simulink library "threeTethers_cl"  (R2018b)
settings: Solver=VariableStepAuto  StartTime=0.0  StopTime=10.0  RelTol=1e-3
undefined symbols (not defined in the file): gnd_station, ini_euler_ang, ini_Rcm_o, R11_g, R1n_cm, R21_g, R2n_cm, R31_g, R3n_cm, rotation_sequence, sim_param
libraries: singleTether_cl x3
settings Model: Creator=mcobb  LastModifiedBy=mcobb

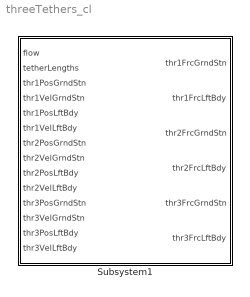
== system threeTethers_cl ==
  Subsystem1 : Subsystem

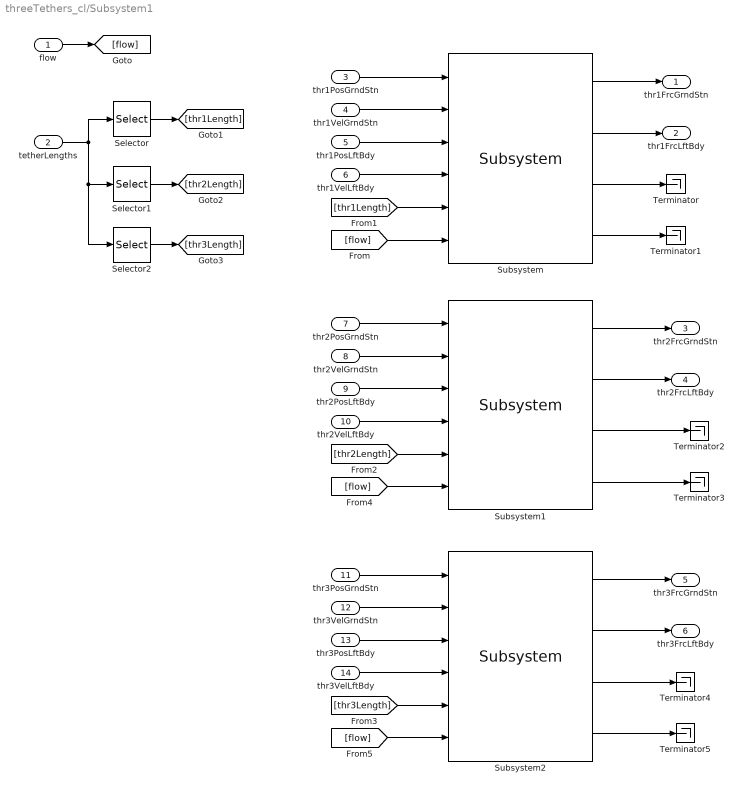
== system threeTethers_cl/Subsystem1 ==
  flow : Inport
  tetherLengths : Inport  Port=2
  thr1PosGrndStn : Inport  Port=3
  thr1VelGrndStn : Inport  Port=4
  thr1PosLftBdy : Inport  Port=5
  thr1VelLftBdy : Inport  Port=6
  thr2PosGrndStn : Inport  Port=7
  thr2VelGrndStn : Inport  Port=8
  thr2PosLftBdy : Inport  Port=9
  thr2VelLftBdy : Inport  Port=10
  thr3PosGrndStn : Inport  Port=11
  thr3VelGrndStn : Inport  Port=12
  thr3PosLftBdy : Inport  Port=13
  thr3VelLftBdy : Inport  Port=14
  Selector : Selector  InputPortWidth=3  IndexOptions=Index vector (dialog)  Indices=1  OutputSizes=1
  Selector1 : Selector  InputPortWidth=3  IndexOptions=Index vector (dialog)  Indices=1  OutputSizes=1
  Selector2 : Selector  InputPortWidth=3  IndexOptions=Index vector (dialog)  Indices=1  OutputSizes=1
  Subsystem : singleTether_cl/Subsystem  N=sim_param.N  dia_t=sim_param.tether_param.tether_diameter(1)  E=sim_param.tether_param.tether_youngs  rho_tether=sim_param.tether_param.tether_density+ sim_param.env_param.density  Cd=sim_param.tether_param.CD_cylinder  zeta=sim_param.tether_param.damping_ratio  rho=sim_param.env_param.density  mass=sim_param.geom_param.mass  ini_Rn_o=ini_Rcm_o + rotation_sequence(ini_euler_ang)*R1n_cm  ini_R1_o=gnd_station + R11_g
  Subsystem1 : singleTether_cl/Subsystem  N=sim_param.N  dia_t=sim_param.tether_param.tether_diameter(2)  E=sim_param.tether_param.tether_youngs  rho_tether=sim_param.tether_param.tether_density+ sim_param.env_param.density  Cd=sim_param.tether_param.CD_cylinder  zeta=sim_param.tether_param.damping_ratio  rho=sim_param.env_param.density  mass=sim_param.geom_param.mass  ini_Rn_o=ini_Rcm_o + rotation_sequence(ini_euler_ang)*R2n_cm  ini_R1_o=gnd_station + R21_g
  Subsystem2 : singleTether_cl/Subsystem  N=sim_param.N  dia_t=sim_param.tether_param.tether_diameter(3)  E=sim_param.tether_param.tether_youngs  rho_tether=sim_param.tether_param.tether_density+ sim_param.env_param.density  Cd=sim_param.tether_param.CD_cylinder  zeta=sim_param.tether_param.damping_ratio  rho=sim_param.env_param.density  mass=sim_param.geom_param.mass  ini_Rn_o=ini_Rcm_o + rotation_sequence(ini_euler_ang)*R3n_cm  ini_R1_o=gnd_station + R31_g
  Terminator{,1..5} (6 alike) : Terminator
  thr1FrcGrndStn : Outport
  thr1FrcLftBdy : Outport  Port=2
  thr2FrcGrndStn : Outport  Port=3
  thr2FrcLftBdy : Outport  Port=4
  thr3FrcGrndStn : Outport  Port=5
  thr3FrcLftBdy : Outport  Port=6
  wires:
  thr1PosGrndStn/1 -> Subsystem/1
  thr1VelGrndStn/1 -> Subsystem/2
  thr1VelLftBdy/1 -> Subsystem/4
  thr1PosLftBdy/1 -> Subsystem/3
  flow/1 -> [flow]
  [flow] -> Subsystem/6
  Selector/1 -> [thr1Length]
  tetherLengths/1 -> Selector/1, Selector1/1, Selector2/1
  Selector1/1 -> [thr2Length]
  Selector2/1 -> [thr3Length]
  [thr1Length] -> Subsystem/5
  [thr2Length] -> Subsystem1/5
  [thr3Length] -> Subsystem2/5
  [flow] -> Subsystem1/6
  [flow] -> Subsystem2/6
  thr2PosGrndStn/1 -> Subsystem1/1
  thr2VelGrndStn/1 -> Subsystem1/2
  thr2PosLftBdy/1 -> Subsystem1/3
  thr2VelLftBdy/1 -> Subsystem1/4
  thr3VelLftBdy/1 -> Subsystem2/4
  thr3PosLftBdy/1 -> Subsystem2/3
  thr3VelGrndStn/1 -> Subsystem2/2
  thr3PosGrndStn/1 -> Subsystem2/1
  Subsystem/1 -> thr1FrcGrndStn/1
  Subsystem/2 -> thr1FrcLftBdy/1
  Subsystem/3 -> Terminator/1
  Subsystem/4 -> Terminator1/1
  Subsystem2/4 -> Terminator5/1
  Subsystem2/3 -> Terminator4/1
  Subsystem2/2 -> thr3FrcLftBdy/1
  Subsystem2/1 -> thr3FrcGrndStn/1
  Subsystem1/4 -> Terminator3/1
  Subsystem1/3 -> Terminator2/1
  Subsystem1/2 -> thr2FrcLftBdy/1
  Subsystem1/1 -> thr2FrcGrndStn/1
